simulink model "untitled"  (R2017b)
settings: Solver=FixedStepAuto  StartTime=0.0  StopTime=10.0  FixedStep=0.01  RelTol=1e-3
libraries: simulink x5
settings Model: Creator=Student  LastModifiedBy=Cosmin

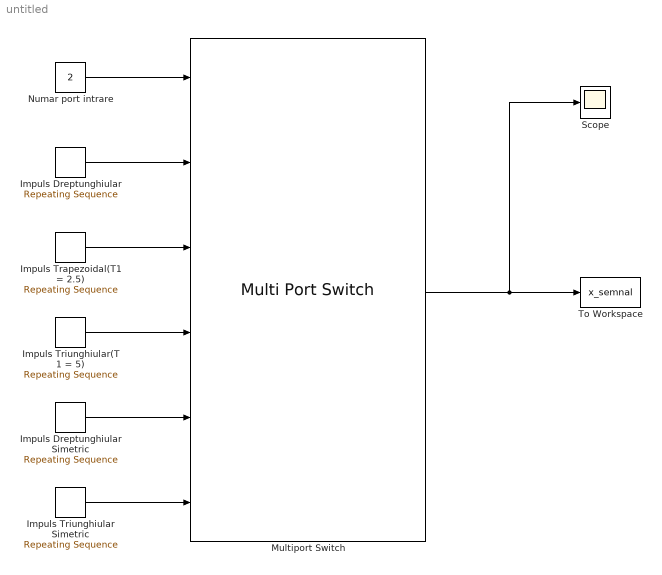
== system untitled ==
  Impuls Dreptunghiular : simulink/Sources/Repeating Sequence  rep_seq_t=[0 0.001 2.5 2.501 5 5.501 7.5 7.501 10 10.001 30]  rep_seq_y=[0 1 1 1 1 1 1 1 1 0 0]
  Impuls Dreptunghiular Simetric : simulink/Sources/Repeating Sequence  rep_seq_t=[0 2]  rep_seq_y=[0 2]
  Impuls Trapezoidal(T1 = 2.5) : simulink/Sources/Repeating Sequence  rep_seq_t=[0 2]  rep_seq_y=[0 2]
  Impuls Triunghiular Simetric : simulink/Sources/Repeating Sequence  rep_seq_t=[0 0.001 2.5 2.501 5 5.501 7.5 7.501 10 10.001 30]  rep_seq_y=[0 0.001 1 0.9996 0 -0.2004 -1 -0.9996 0 0 0]
  Impuls Triunghiular(T1 = 5) : simulink/Sources/Repeating Sequence  rep_seq_t=[0 2]  rep_seq_y=[0 2]
  Multiport Switch : MultiPortSwitch  Inputs=5
  Numar port intrare : Constant  Value=2
  Scope : Scope
  To Workspace : ToWorkspace  VariableName=x_semnal  SaveFormat=Timeseries  SampleTime=-1
  wires:
  Numar port intrare/1 -> Multiport Switch/1
  Impuls Dreptunghiular/1 -> Multiport Switch/2
  Impuls Trapezoidal(T1 = 2.5)/1 -> Multiport Switch/3
  Impuls Triunghiular(T1 = 5)/1 -> Multiport Switch/4
  Impuls Dreptunghiular Simetric/1 -> Multiport Switch/5
  Impuls Triunghiular Simetric/1 -> Multiport Switch/6
  Multiport Switch/1 -> Scope/1, To Workspace/1
